simulink model "Q7Speed_Controller"  (R2013a)
settings: Solver=ode45  StartTime=0.0  StopTime=5  MaxStep=1e-4  RelTol=1e-3
libraries: simulink x1
settings Model: Creator=Sony  LastModifiedBy=Sony

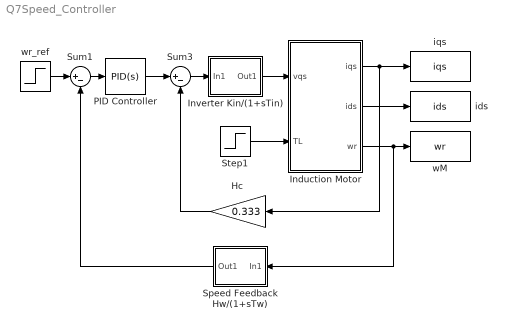
== system Q7Speed_Controller ==
  Hc : Gain  Gain=0.333
  Induction Motor : Subsystem  mask{Rs=0.277, Lr=0.05606, Ls=0.0553, Lm=0.0538, La=0.0553-((0.0538*0.0538)/0.05606), J=0.0165, B=0.05, ws=2*pi*60, P=4}
      mask prompts: Rs "Rs (ohm)"; Lr "Lr (H)"; Ls "Ls (H)"; Lm "Lm (H)"; La "La (H)"; J "J (kgm^2)"; B "B (kgm^2/s)"; ws "ws (rad/s)"
  Inverter Kin/(1+sTin) : Subsystem  mask{Kin=1, Tin=1/(2*2000)}
  PID Controller : simulink/Continuous/PID Controller  Controller=PID  TimeDomain=Continuous-time  SampleTime=1  IntegratorMethod=Forward Euler  FilterMethod=Forward Euler  Form=Parallel  P=0.2  I=0.1  D=0  N=100  InitialConditionSource=internal  InitialConditionForIntegrator=0  InitialConditionForFilter=0  ExternalReset=none  LimitOutput=off  UpperSaturationLimit=inf  LowerSaturationLimit=-inf  LinearizeAsGain=on  AntiWindupMode=none  Kb=1  TrackingMode=off  Kt=1  PParamMin=[]  PParamMax=[]  IParamMin=[]  IParamMax=[]  DParamMin=[]  DParamMax=[]  NParamMin=[]  NParamMax=[]  KbParamMin=[]  KbParamMax=[]  KtParamMin=[]  KtParamMax=[]  POutMin=[]  POutMax=[]  IOutMin=[]  IOutMax=[]  DOutMin=[]  DOutMax=[]  NOutMin=[]  NOutMax=[]  KbOutMin=[]  KbOutMax=[]  KtOutMin=[]  KtOutMax=[]  IntegratorOutMin=[]  IntegratorOutMax=[]  FilterOutMin=[]  FilterOutMax=[]  SumOutMin=[]  SumOutMax=[]  SumI1OutMin=[]  SumI1OutMax=[]  SumI2OutMin=[]  SumI2OutMax=[]  SumI3OutMin=[]  SumI3OutMax=[]  SumDOutMin=[]  SumDOutMax=[]  SaturationOutMin=[]  SaturationOutMax=[]  IntegratorContinuousStateAttributes=''  IntegratorStateMustResolveToSignalObject=off  IntegratorRTWStateStorageClass=Auto  FilterContinuousStateAttributes=''  FilterStateMustResolveToSignalObject=off  FilterRTWStateStorageClass=Auto
  Speed Feedback Hw/(1+sTw) : Subsystem  mask{Hw=1, Tw=0.002}
  Step1 : Step  Time=2.5  SampleTime=0
  Sum1 : Sum  Inputs=|+-
  Sum3 : Sum  Inputs=|+-
  ids : ToWorkspace  VariableName=ids  SampleTime=-1  SaveFormat=Timeseries
  iqs : ToWorkspace  VariableName=iqs  SampleTime=-1  SaveFormat=Timeseries
  wM : ToWorkspace  VariableName=wr  SampleTime=-1  SaveFormat=Timeseries
  wr_ref : Step  Time=0.1  After=100  SampleTime=0
  wires:
  Induction Motor/1(iqs) -> Hc/1, iqs/1
  Induction Motor/3(wr) -> Speed Feedback Hw/(1+sTw)/1(In1), wM/1
  Inverter Kin/(1+sTin)/1(Out1) -> Induction Motor/1(vqs)
  Step1/1 -> Induction Motor/2(TL)
  Induction Motor/2(ids) -> ids/1
  Hc/1 -> Sum3/2
  Sum3/1 -> Inverter Kin/(1+sTin)/1(In1)
  PID Controller/1 -> Sum3/1
  Speed Feedback Hw/(1+sTw)/1(Out1) -> Sum1/2
  wr_ref/1 -> Sum1/1
  Sum1/1 -> PID Controller/1

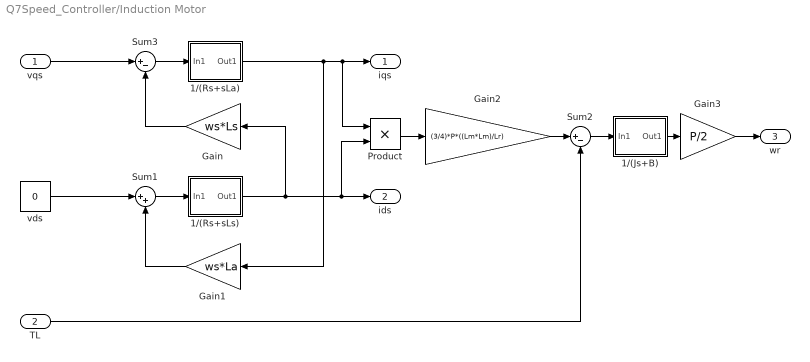
== system Q7Speed_Controller/Induction Motor ==
  vqs : Inport
  TL : Inport  Port=2
  1/(Js+B) : Subsystem  mask{J=J, B=B}
  1/(Rs+sLa) : Subsystem  mask{L=La, R=Rs}
      mask prompts: L "L (Henry)"; R "R (Ohm)"
  1/(Rs+sLs) : Subsystem  mask{L=Ls, R=Rs}
      mask prompts: L "L (Henry)"; R "R (Ohm)"
  Gain : Gain  Gain=ws*Ls
  Gain1 : Gain  Gain=ws*La
  Gain2 : Gain  Gain=(3/4)*P*((Lm*Lm)/Lr)
  Gain3 : Gain  Gain=P/2
  Product : Product
  Sum1 : Sum  Inputs=|++
  Sum2 : Sum  Inputs=|+-
  Sum3 : Sum  Inputs=|+-
  vds : Constant  Value=0
  iqs : Outport
  ids : Outport  Port=2
  wr : Outport  Port=3
  wires:
  vqs/1 -> Sum3/1
  1/(Rs+sLs)/1(Out1) -> Gain/1, Product/2, ids/1
  Gain/1 -> Sum3/2
  vds/1 -> Sum1/1
  1/(Rs+sLa)/1(Out1) -> Gain1/1, Product/1, iqs/1
  Gain1/1 -> Sum1/2
  Sum3/1 -> 1/(Rs+sLa)/1(In1)
  Sum1/1 -> 1/(Rs+sLs)/1(In1)
  Product/1 -> Gain2/1
  Gain2/1 -> Sum2/1
  TL/1 -> Sum2/2
  Sum2/1 -> 1/(Js+B)/1(In1)
  1/(Js+B)/1(Out1) -> Gain3/1
  Gain3/1 -> wr/1

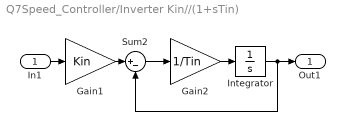
== system Q7Speed_Controller/Inverter Kin//(1+sTin) ==
  In1 : Inport
  Gain1 : Gain  Gain=Kin
  Gain2 : Gain  Gain=1/Tin
  Integrator : Integrator
  Sum2 : Sum  Inputs=|+-
  Out1 : Outport
  wires:
  Integrator/1 -> Sum2/2, Out1/1
  Sum2/1 -> Gain2/1
  Gain2/1 -> Integrator/1
  In1/1 -> Gain1/1
  Gain1/1 -> Sum2/1

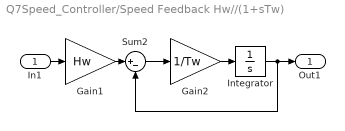
== system Q7Speed_Controller/Speed Feedback Hw//(1+sTw) ==
  In1 : Inport
  Gain1 : Gain  Gain=Hw
  Gain2 : Gain  Gain=1/Tw
  Integrator : Integrator
  Sum2 : Sum  Inputs=|+-
  Out1 : Outport
  wires:
  Integrator/1 -> Sum2/2, Out1/1
  Sum2/1 -> Gain2/1
  Gain2/1 -> Integrator/1
  In1/1 -> Gain1/1
  Gain1/1 -> Sum2/1

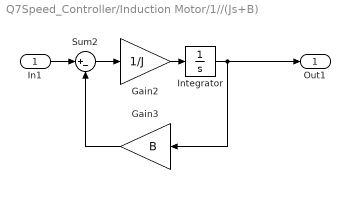
== system Q7Speed_Controller/Induction Motor/1//(Js+B) ==
  In1 : Inport
  Gain2 : Gain  Gain=1/J
  Gain3 : Gain  Gain=B
  Integrator : Integrator
  Sum2 : Sum  Inputs=|+-
  Out1 : Outport
  wires:
  Gain3/1 -> Sum2/2
  Sum2/1 -> Gain2/1
  Gain2/1 -> Integrator/1
  In1/1 -> Sum2/1
  Integrator/1 -> Out1/1, Gain3/1

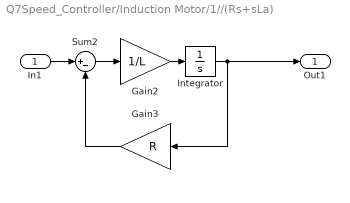
== system Q7Speed_Controller/Induction Motor/1//(Rs+sLa) ==
  In1 : Inport
  Gain2 : Gain  Gain=1/L
  Gain3 : Gain  Gain=R
  Integrator : Integrator
  Sum2 : Sum  Inputs=|+-
  Out1 : Outport
  wires:
  Gain3/1 -> Sum2/2
  Sum2/1 -> Gain2/1
  Gain2/1 -> Integrator/1
  In1/1 -> Sum2/1
  Integrator/1 -> Out1/1, Gain3/1

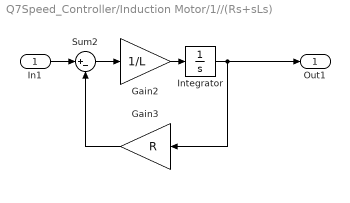
== system Q7Speed_Controller/Induction Motor/1//(Rs+sLs) ==
  In1 : Inport
  Gain2 : Gain  Gain=1/L
  Gain3 : Gain  Gain=R
  Integrator : Integrator
  Sum2 : Sum  Inputs=|+-
  Out1 : Outport
  wires:
  Gain3/1 -> Sum2/2
  Sum2/1 -> Gain2/1
  Gain2/1 -> Integrator/1
  In1/1 -> Sum2/1
  Integrator/1 -> Out1/1, Gain3/1
